simulink model "lab2_second_part"  (R2022a)
settings: Solver=VariableStepAuto  StartTime=0.0  StopTime=10.0  RelTol=1e-3
settings Model: Creator=Даниил  LastModifiedBy=Даниил

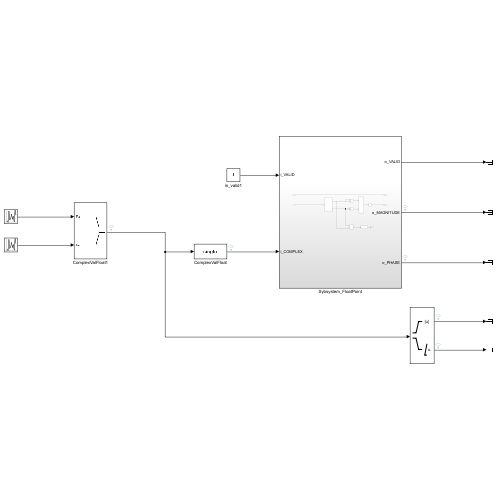
[thumbnail: Simulink's stored preview of the top-level diagram]
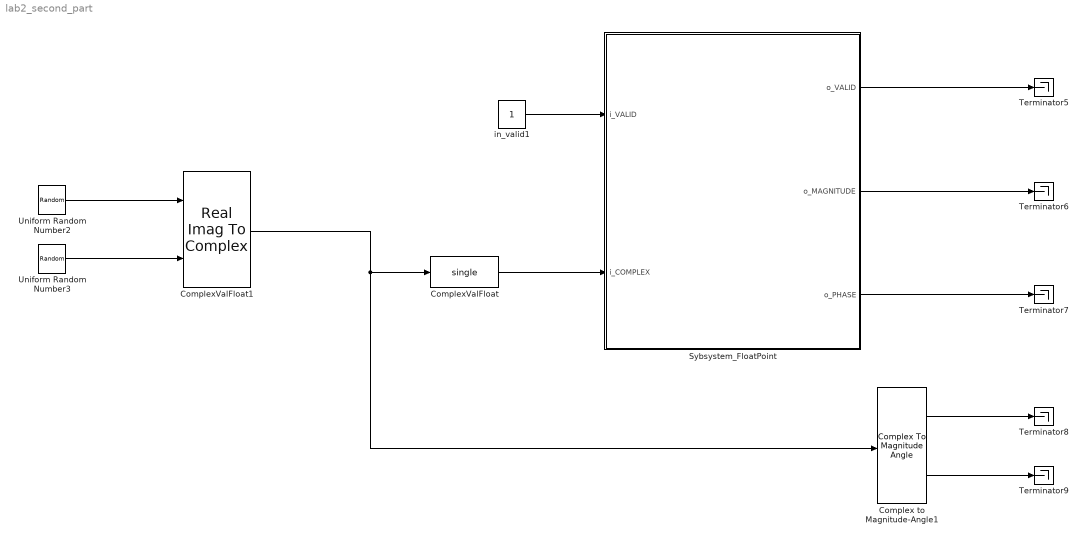
== system lab2_second_part ==
  Complex to Magnitude-Angle1 : ComplexToMagnitudeAngle
  ComplexValFloat : DataTypeConversion  OutDataTypeStr=single  RndMeth=Round  SaturateOnIntegerOverflow=off
  ComplexValFloat1 : RealImagToComplex
  Sybsystem_FloatPoint : Subsystem
  Terminator{5..9} (5 alike) : Terminator
  Uniform Random Number2 : UniformRandomNumber  Minimum=-2 ^(17 - 1)  Maximum=2 ^(17-1) - 1  Seed=17  SampleTime=1
  Uniform Random Number3 : UniformRandomNumber  Minimum=-2 ^(17 - 1)  Maximum=2 ^(17-1) - 1  Seed=18  SampleTime=1
  in_valid1 : Constant  OutDataTypeStr=boolean  SampleTime=1
  wires:
  ComplexValFloat/1 -> Sybsystem_FloatPoint/2(i_COMPLEX)
  Complex to Magnitude-Angle1/1 -> Terminator8/1
  Uniform Random Number3/1 -> ComplexValFloat1/2
  Sybsystem_FloatPoint/1(o_VALID) -> Terminator5/1
  Complex to Magnitude-Angle1/2 -> Terminator9/1
  Sybsystem_FloatPoint/2(o_MAGNITUDE) -> Terminator6/1
  Uniform Random Number2/1 -> ComplexValFloat1/1
  in_valid1/1 -> Sybsystem_FloatPoint/1(i_VALID)
  Sybsystem_FloatPoint/3(o_PHASE) -> Terminator7/1
  ComplexValFloat1/1 -> Complex to Magnitude-Angle1/1, ComplexValFloat/1

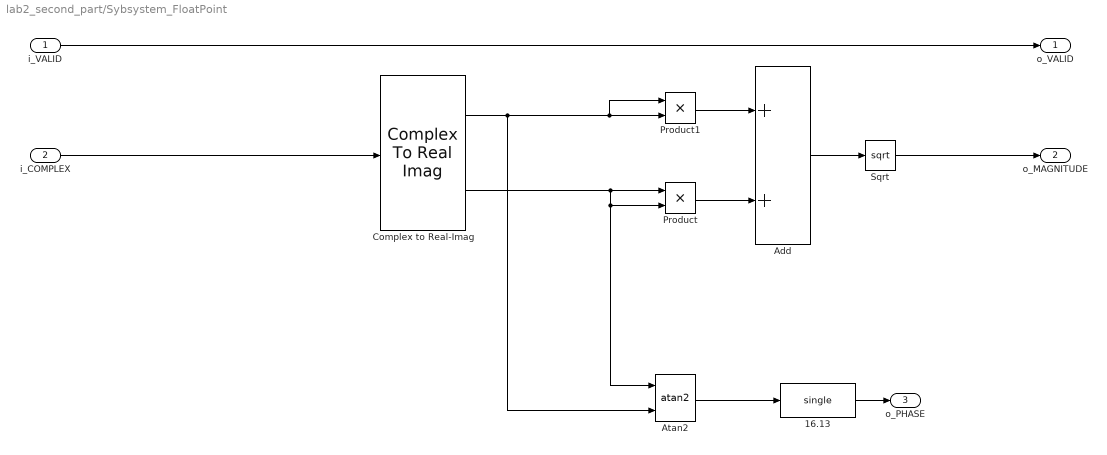
== system lab2_second_part/Sybsystem_FloatPoint ==
  i_VALID : Inport  OutDataTypeStr=boolean
  i_COMPLEX : Inport  Port=2
  16.13 : DataTypeConversion  OutDataTypeStr=single  RndMeth=Round  SaturateOnIntegerOverflow=off
  Add : Sum
  Atan2 : Trigonometry  Operator=atan2  ApproximationMethod=CORDIC
  Complex to Real-Imag : ComplexToRealImag
  Product : Product
  Product1 : Product
  Sqrt : Sqrt  OutDataTypeStr=single
  o_VALID : Outport
  o_MAGNITUDE : Outport  Port=2
  o_PHASE : Outport  Port=3
  wires:
  Add/1 -> Sqrt/1
  Product1/1 -> Add/1
  Sqrt/1 -> o_MAGNITUDE/1
  Product/1 -> Add/2
  Atan2/1 -> 16.13/1
  i_COMPLEX/1 -> Complex to Real-Imag/1
  i_VALID/1 -> o_VALID/1
  16.13/1 -> o_PHASE/1
  Complex to Real-Imag/2 -> Atan2/1, Product/2, Product/1
  Complex to Real-Imag/1 -> Product1/1, Product1/2, Atan2/2
